simulink model "sim_sys2"  (R2013b)
settings: Solver=ode45  StartTime=0.0  StopTime=5000  RelTol=1e-3
undefined symbols (not defined in the file or in its folder): msdft_comb, resonator, sys_lib, twiddle_factors
libraries: xbsIndex_r4 x3996, casper_library_misc x310, xps_library x1
(part 5 of 46)

== system sim_sys2/Subsystem/resonator37 ==
  note: No estoy tan seguro
      | de este delay....
  din : Inport
  sync : Inport  Port=2
  rst : Inport  Port=3
  Delay{,1..2,4} (4 alike) : xbsIndex_r4/Delay  rst=off  infoeditControl=Selection of Reset will increase slice count due to use of real FFs and instead of SRLs  en=off  latency=1  dbl_ovrd=off  reg_retiming=off  block_type=delay
  Delay3 : xbsIndex_r4/Delay  rst=off  infoeditControl=Selection of Reset will increase slice count due to use of real FFs and instead of SRLs  en=off  latency=5  dbl_ovrd=off  reg_retiming=off  block_type=delay
  cmult : Subsystem  AncestorBlock=casper_library_multipliers/cmult  mask(cmult){n_bits_a=input_bitsize, bin_pt_a=input_frac, n_bits_b=twid_bitsize, bin_pt_b=twid_bitsize-2, n_bits_ab=input_bitsize+twid_bitsize+1, bin_pt_ab=input_frac+twid_bitsize-2, quantization=Truncate, overflow=Wrap, in_latency=0, mult_latency=3, add_latency=1, conv_latency=1, conjugated=off, async=off, pipelined_enable=on, multiplier_implementation=behavioral HDL}
      mask prompts: n_bits_a "Number of Bits 'a'"; bin_pt_a "Binary Point 'a'"; n_bits_b "Number of Bits 'b'"; bin_pt_b "Binary Point 'b'"; n_bits_ab "Number of Bits 'ab'"; bin_pt_ab "Binary Point 'ab'"; in_latency "Input latency"; mult_latency "Multiplier Latency"; add_latency "Adder Latency"; conv_latency "Convert latency"; conjugated "Conjugate"; async "asynchronous operation"; pipelined_enable "enable pipeline"; multiplier_implementation "Multiplier implementation"
      mask help:
      | Multiplies two complex numbers using 4 multipliers and 2 adders.
      | Conjugation is optional.
      mask init: same as sim_sys2/Subsystem/resonator/cmult
      settings: AttributesFormatString=|
      | 11_9 * 15_13 ==> 27_22
      | Truncate, Wrap
      | Latency=0
      mask TypeOptions quantization: Truncate | Round  (unbiased: +/- Inf) | Round  (unbiased: Even Values)
      mask TypeOptions overflow: Wrap | Saturate | Flag as error
      mask TypeOptions multiplier_implementation: behavioral HDL | standard core | embedded multiplier core
  complex_conj : Subsystem  AncestorBlock=casper_library_misc/complex_conj  mask(complex_conj){n_inputs=1, n_bits=twid_bitsize, bin_pt=twid_bitsize-2, latency=1, overflow=Wrap}
      mask prompts: n_inputs "number simultaneous inputs"; n_bits "input bitwidth"; bin_pt "input binary point"; overflow "overflow strategy"
      mask help: Finds the complex conjugate of complex inputs.
      mask init:
      | complex_conj_init(gcb, ...
      |     'n_inputs', n_inputs, ...
      |     'n_bits', n_bits, ...
      |     'bin_pt', bin_pt, ...
      |     'latency', latency, ...
      |     'overflow', overflow);
      mask TypeOptions overflow: Wrap | Saturate | Flag as error
  complex_sum : Subsystem  mask(complex_sum){a_bitsize=input_bitsize+twid_bitsize+1, a_frac=input_frac+twid_bitsize-2, b_bitsize=res_bitsize, b_frac=input_frac+twid_bitsize-2, out_bitsize=res_bitsize, latency=add_lat}
      mask prompts: out_bitsize "output_bitsize"
      mask init: same as sim_sys2/Subsystem/resonator/complex_sum
      settings: AttributesFormatString=latency=0
  twiddle : Subsystem  mask(msdft_twiddle_factors){fft_len=fft_len, bin_num=bin_number, twid_bitsize=twid_bitsize}
      mask prompts: fft_len "fft_len(2^)"; bin_num "bin number"; twid_bitsize "twiddle bitsize"
      mask init:
      | twid_msdft_init(gcb, ...
      |         'fft_len', fft_len, ...
      |         'bin_num', bin_num, ...
      |         'twid_bitsize', twid_bitsize)
      settings: AttributesFormatString=N=10, k=87
  Out1 : Outport
  twidd : Outport  Port=2
  wires:
  Delay4/1 -> twidd/1
  Delay3/1 -> Delay4/1
  Delay1/1 -> Delay3/1
  Delay2/1 -> complex_sum/2(b)
  complex_sum/1(dout) -> Out1/1, Delay2/1
  cmult/1(ab) -> complex_sum/1(a)
  Delay/1 -> cmult/1(a)
  complex_conj/1(z*) -> cmult/2(b)
  twiddle/1(dout) -> Delay1/1, complex_conj/1(z)
  din/1 -> Delay/1
  rst/1 -> twiddle/2(rst)
  sync/1 -> twiddle/1(sync)

== system sim_sys2/Subsystem/resonator38 ==
  note: No estoy tan seguro
      | de este delay....
  din : Inport
  sync : Inport  Port=2
  rst : Inport  Port=3
  Delay{,1..2,4} (4 alike) : xbsIndex_r4/Delay  rst=off  infoeditControl=Selection of Reset will increase slice count due to use of real FFs and instead of SRLs  en=off  latency=1  dbl_ovrd=off  reg_retiming=off  block_type=delay
  Delay3 : xbsIndex_r4/Delay  rst=off  infoeditControl=Selection of Reset will increase slice count due to use of real FFs and instead of SRLs  en=off  latency=5  dbl_ovrd=off  reg_retiming=off  block_type=delay
  cmult : Subsystem  AncestorBlock=casper_library_multipliers/cmult  mask(cmult){n_bits_a=input_bitsize, bin_pt_a=input_frac, n_bits_b=twid_bitsize, bin_pt_b=twid_bitsize-2, n_bits_ab=input_bitsize+twid_bitsize+1, bin_pt_ab=input_frac+twid_bitsize-2, quantization=Truncate, overflow=Wrap, in_latency=0, mult_latency=3, add_latency=1, conv_latency=1, conjugated=off, async=off, pipelined_enable=on, multiplier_implementation=behavioral HDL}
      mask prompts: n_bits_a "Number of Bits 'a'"; bin_pt_a "Binary Point 'a'"; n_bits_b "Number of Bits 'b'"; bin_pt_b "Binary Point 'b'"; n_bits_ab "Number of Bits 'ab'"; bin_pt_ab "Binary Point 'ab'"; in_latency "Input latency"; mult_latency "Multiplier Latency"; add_latency "Adder Latency"; conv_latency "Convert latency"; conjugated "Conjugate"; async "asynchronous operation"; pipelined_enable "enable pipeline"; multiplier_implementation "Multiplier implementation"
      mask help:
      | Multiplies two complex numbers using 4 multipliers and 2 adders.
      | Conjugation is optional.
      mask init: same as sim_sys2/Subsystem/resonator/cmult
      settings: AttributesFormatString=|
      | 11_9 * 15_13 ==> 27_22
      | Truncate, Wrap
      | Latency=0
      mask TypeOptions quantization: Truncate | Round  (unbiased: +/- Inf) | Round  (unbiased: Even Values)
      mask TypeOptions overflow: Wrap | Saturate | Flag as error
      mask TypeOptions multiplier_implementation: behavioral HDL | standard core | embedded multiplier core
  complex_conj : Subsystem  AncestorBlock=casper_library_misc/complex_conj  mask(complex_conj){n_inputs=1, n_bits=twid_bitsize, bin_pt=twid_bitsize-2, latency=1, overflow=Wrap}
      mask prompts: n_inputs "number simultaneous inputs"; n_bits "input bitwidth"; bin_pt "input binary point"; overflow "overflow strategy"
      mask help: Finds the complex conjugate of complex inputs.
      mask init:
      | complex_conj_init(gcb, ...
      |     'n_inputs', n_inputs, ...
      |     'n_bits', n_bits, ...
      |     'bin_pt', bin_pt, ...
      |     'latency', latency, ...
      |     'overflow', overflow);
      mask TypeOptions overflow: Wrap | Saturate | Flag as error
  complex_sum : Subsystem  mask(complex_sum){a_bitsize=input_bitsize+twid_bitsize+1, a_frac=input_frac+twid_bitsize-2, b_bitsize=res_bitsize, b_frac=input_frac+twid_bitsize-2, out_bitsize=res_bitsize, latency=add_lat}
      mask prompts: out_bitsize "output_bitsize"
      mask init: same as sim_sys2/Subsystem/resonator/complex_sum
      settings: AttributesFormatString=latency=0
  twiddle : Subsystem  mask(msdft_twiddle_factors){fft_len=fft_len, bin_num=bin_number, twid_bitsize=twid_bitsize}
      mask prompts: fft_len "fft_len(2^)"; bin_num "bin number"; twid_bitsize "twiddle bitsize"
      mask init:
      | twid_msdft_init(gcb, ...
      |         'fft_len', fft_len, ...
      |         'bin_num', bin_num, ...
      |         'twid_bitsize', twid_bitsize)
      settings: AttributesFormatString=N=10, k=88
  Out1 : Outport
  twidd : Outport  Port=2
  wires:
  Delay4/1 -> twidd/1
  Delay3/1 -> Delay4/1
  Delay1/1 -> Delay3/1
  Delay2/1 -> complex_sum/2(b)
  complex_sum/1(dout) -> Out1/1, Delay2/1
  cmult/1(ab) -> complex_sum/1(a)
  Delay/1 -> cmult/1(a)
  complex_conj/1(z*) -> cmult/2(b)
  twiddle/1(dout) -> Delay1/1, complex_conj/1(z)
  din/1 -> Delay/1
  rst/1 -> twiddle/2(rst)
  sync/1 -> twiddle/1(sync)

== system sim_sys2/Subsystem/resonator39 ==
  note: No estoy tan seguro
      | de este delay....
  din : Inport
  sync : Inport  Port=2
  rst : Inport  Port=3
  Delay{,1..2,4} (4 alike) : xbsIndex_r4/Delay  rst=off  infoeditControl=Selection of Reset will increase slice count due to use of real FFs and instead of SRLs  en=off  latency=1  dbl_ovrd=off  reg_retiming=off  block_type=delay
  Delay3 : xbsIndex_r4/Delay  rst=off  infoeditControl=Selection of Reset will increase slice count due to use of real FFs and instead of SRLs  en=off  latency=5  dbl_ovrd=off  reg_retiming=off  block_type=delay
  cmult : Subsystem  AncestorBlock=casper_library_multipliers/cmult  mask(cmult){n_bits_a=input_bitsize, bin_pt_a=input_frac, n_bits_b=twid_bitsize, bin_pt_b=twid_bitsize-2, n_bits_ab=input_bitsize+twid_bitsize+1, bin_pt_ab=input_frac+twid_bitsize-2, quantization=Truncate, overflow=Wrap, in_latency=0, mult_latency=3, add_latency=1, conv_latency=1, conjugated=off, async=off, pipelined_enable=on, multiplier_implementation=behavioral HDL}
      mask prompts: n_bits_a "Number of Bits 'a'"; bin_pt_a "Binary Point 'a'"; n_bits_b "Number of Bits 'b'"; bin_pt_b "Binary Point 'b'"; n_bits_ab "Number of Bits 'ab'"; bin_pt_ab "Binary Point 'ab'"; in_latency "Input latency"; mult_latency "Multiplier Latency"; add_latency "Adder Latency"; conv_latency "Convert latency"; conjugated "Conjugate"; async "asynchronous operation"; pipelined_enable "enable pipeline"; multiplier_implementation "Multiplier implementation"
      mask help:
      | Multiplies two complex numbers using 4 multipliers and 2 adders.
      | Conjugation is optional.
      mask init: same as sim_sys2/Subsystem/resonator/cmult
      settings: AttributesFormatString=|
      | 11_9 * 15_13 ==> 27_22
      | Truncate, Wrap
      | Latency=0
      mask TypeOptions quantization: Truncate | Round  (unbiased: +/- Inf) | Round  (unbiased: Even Values)
      mask TypeOptions overflow: Wrap | Saturate | Flag as error
      mask TypeOptions multiplier_implementation: behavioral HDL | standard core | embedded multiplier core
  complex_conj : Subsystem  AncestorBlock=casper_library_misc/complex_conj  mask(complex_conj){n_inputs=1, n_bits=twid_bitsize, bin_pt=twid_bitsize-2, latency=1, overflow=Wrap}
      mask prompts: n_inputs "number simultaneous inputs"; n_bits "input bitwidth"; bin_pt "input binary point"; overflow "overflow strategy"
      mask help: Finds the complex conjugate of complex inputs.
      mask init:
      | complex_conj_init(gcb, ...
      |     'n_inputs', n_inputs, ...
      |     'n_bits', n_bits, ...
      |     'bin_pt', bin_pt, ...
      |     'latency', latency, ...
      |     'overflow', overflow);
      mask TypeOptions overflow: Wrap | Saturate | Flag as error
  complex_sum : Subsystem  mask(complex_sum){a_bitsize=input_bitsize+twid_bitsize+1, a_frac=input_frac+twid_bitsize-2, b_bitsize=res_bitsize, b_frac=input_frac+twid_bitsize-2, out_bitsize=res_bitsize, latency=add_lat}
      mask prompts: out_bitsize "output_bitsize"
      mask init: same as sim_sys2/Subsystem/resonator/complex_sum
      settings: AttributesFormatString=latency=0
  twiddle : Subsystem  mask(msdft_twiddle_factors){fft_len=fft_len, bin_num=bin_number, twid_bitsize=twid_bitsize}
      mask prompts: fft_len "fft_len(2^)"; bin_num "bin number"; twid_bitsize "twiddle bitsize"
      mask init:
      | twid_msdft_init(gcb, ...
      |         'fft_len', fft_len, ...
      |         'bin_num', bin_num, ...
      |         'twid_bitsize', twid_bitsize)
      settings: AttributesFormatString=N=10, k=89
  Out1 : Outport
  twidd : Outport  Port=2
  wires:
  Delay4/1 -> twidd/1
  Delay3/1 -> Delay4/1
  Delay1/1 -> Delay3/1
  Delay2/1 -> complex_sum/2(b)
  complex_sum/1(dout) -> Out1/1, Delay2/1
  cmult/1(ab) -> complex_sum/1(a)
  Delay/1 -> cmult/1(a)
  complex_conj/1(z*) -> cmult/2(b)
  twiddle/1(dout) -> Delay1/1, complex_conj/1(z)
  din/1 -> Delay/1
  rst/1 -> twiddle/2(rst)
  sync/1 -> twiddle/1(sync)

== system sim_sys2/Subsystem/resonator4 ==
  note: No estoy tan seguro
      | de este delay....
  din : Inport
  sync : Inport  Port=2
  rst : Inport  Port=3
  Delay{,1..2,4} (4 alike) : xbsIndex_r4/Delay  rst=off  infoeditControl=Selection of Reset will increase slice count due to use of real FFs and instead of SRLs  en=off  latency=1  dbl_ovrd=off  reg_retiming=off  block_type=delay
  Delay3 : xbsIndex_r4/Delay  rst=off  infoeditControl=Selection of Reset will increase slice count due to use of real FFs and instead of SRLs  en=off  latency=5  dbl_ovrd=off  reg_retiming=off  block_type=delay
  cmult : Subsystem  AncestorBlock=casper_library_multipliers/cmult  mask(cmult){n_bits_a=input_bitsize, bin_pt_a=input_frac, n_bits_b=twid_bitsize, bin_pt_b=twid_bitsize-2, n_bits_ab=input_bitsize+twid_bitsize+1, bin_pt_ab=input_frac+twid_bitsize-2, quantization=Truncate, overflow=Wrap, in_latency=0, mult_latency=3, add_latency=1, conv_latency=1, conjugated=off, async=off, pipelined_enable=on, multiplier_implementation=behavioral HDL}
      mask prompts: n_bits_a "Number of Bits 'a'"; bin_pt_a "Binary Point 'a'"; n_bits_b "Number of Bits 'b'"; bin_pt_b "Binary Point 'b'"; n_bits_ab "Number of Bits 'ab'"; bin_pt_ab "Binary Point 'ab'"; in_latency "Input latency"; mult_latency "Multiplier Latency"; add_latency "Adder Latency"; conv_latency "Convert latency"; conjugated "Conjugate"; async "asynchronous operation"; pipelined_enable "enable pipeline"; multiplier_implementation "Multiplier implementation"
      mask help:
      | Multiplies two complex numbers using 4 multipliers and 2 adders.
      | Conjugation is optional.
      mask init: same as sim_sys2/Subsystem/resonator/cmult
      settings: AttributesFormatString=|
      | 11_9 * 15_13 ==> 27_22
      | Truncate, Wrap
      | Latency=0
      mask TypeOptions quantization: Truncate | Round  (unbiased: +/- Inf) | Round  (unbiased: Even Values)
      mask TypeOptions overflow: Wrap | Saturate | Flag as error
      mask TypeOptions multiplier_implementation: behavioral HDL | standard core | embedded multiplier core
  complex_conj : Subsystem  AncestorBlock=casper_library_misc/complex_conj  mask(complex_conj){n_inputs=1, n_bits=twid_bitsize, bin_pt=twid_bitsize-2, latency=1, overflow=Wrap}
      mask prompts: n_inputs "number simultaneous inputs"; n_bits "input bitwidth"; bin_pt "input binary point"; overflow "overflow strategy"
      mask help: Finds the complex conjugate of complex inputs.
      mask init:
      | complex_conj_init(gcb, ...
      |     'n_inputs', n_inputs, ...
      |     'n_bits', n_bits, ...
      |     'bin_pt', bin_pt, ...
      |     'latency', latency, ...
      |     'overflow', overflow);
      mask TypeOptions overflow: Wrap | Saturate | Flag as error
  complex_sum : Subsystem  mask(complex_sum){a_bitsize=input_bitsize+twid_bitsize+1, a_frac=input_frac+twid_bitsize-2, b_bitsize=res_bitsize, b_frac=input_frac+twid_bitsize-2, out_bitsize=res_bitsize, latency=add_lat}
      mask prompts: out_bitsize "output_bitsize"
      mask init: same as sim_sys2/Subsystem/resonator/complex_sum
      settings: AttributesFormatString=latency=0
  twiddle : Subsystem  mask(msdft_twiddle_factors){fft_len=fft_len, bin_num=bin_number, twid_bitsize=twid_bitsize}
      mask prompts: fft_len "fft_len(2^)"; bin_num "bin number"; twid_bitsize "twiddle bitsize"
      mask init:
      | twid_msdft_init(gcb, ...
      |         'fft_len', fft_len, ...
      |         'bin_num', bin_num, ...
      |         'twid_bitsize', twid_bitsize)
      settings: AttributesFormatString=N=10, k=54
  Out1 : Outport
  twidd : Outport  Port=2
  wires:
  Delay4/1 -> twidd/1
  Delay3/1 -> Delay4/1
  Delay1/1 -> Delay3/1
  Delay2/1 -> complex_sum/2(b)
  complex_sum/1(dout) -> Out1/1, Delay2/1
  cmult/1(ab) -> complex_sum/1(a)
  Delay/1 -> cmult/1(a)
  complex_conj/1(z*) -> cmult/2(b)
  twiddle/1(dout) -> Delay1/1, complex_conj/1(z)
  din/1 -> Delay/1
  rst/1 -> twiddle/2(rst)
  sync/1 -> twiddle/1(sync)

== system sim_sys2/Subsystem/resonator40 ==
  note: No estoy tan seguro
      | de este delay....
  din : Inport
  sync : Inport  Port=2
  rst : Inport  Port=3
  Delay{,1..2,4} (4 alike) : xbsIndex_r4/Delay  rst=off  infoeditControl=Selection of Reset will increase slice count due to use of real FFs and instead of SRLs  en=off  latency=1  dbl_ovrd=off  reg_retiming=off  block_type=delay
  Delay3 : xbsIndex_r4/Delay  rst=off  infoeditControl=Selection of Reset will increase slice count due to use of real FFs and instead of SRLs  en=off  latency=5  dbl_ovrd=off  reg_retiming=off  block_type=delay
  cmult : Subsystem  AncestorBlock=casper_library_multipliers/cmult  mask(cmult){n_bits_a=input_bitsize, bin_pt_a=input_frac, n_bits_b=twid_bitsize, bin_pt_b=twid_bitsize-2, n_bits_ab=input_bitsize+twid_bitsize+1, bin_pt_ab=input_frac+twid_bitsize-2, quantization=Truncate, overflow=Wrap, in_latency=0, mult_latency=3, add_latency=1, conv_latency=1, conjugated=off, async=off, pipelined_enable=on, multiplier_implementation=behavioral HDL}
      mask prompts: n_bits_a "Number of Bits 'a'"; bin_pt_a "Binary Point 'a'"; n_bits_b "Number of Bits 'b'"; bin_pt_b "Binary Point 'b'"; n_bits_ab "Number of Bits 'ab'"; bin_pt_ab "Binary Point 'ab'"; in_latency "Input latency"; mult_latency "Multiplier Latency"; add_latency "Adder Latency"; conv_latency "Convert latency"; conjugated "Conjugate"; async "asynchronous operation"; pipelined_enable "enable pipeline"; multiplier_implementation "Multiplier implementation"
      mask help:
      | Multiplies two complex numbers using 4 multipliers and 2 adders.
      | Conjugation is optional.
      mask init: same as sim_sys2/Subsystem/resonator/cmult
      settings: AttributesFormatString=|
      | 11_9 * 15_13 ==> 27_22
      | Truncate, Wrap
      | Latency=0
      mask TypeOptions quantization: Truncate | Round  (unbiased: +/- Inf) | Round  (unbiased: Even Values)
      mask TypeOptions overflow: Wrap | Saturate | Flag as error
      mask TypeOptions multiplier_implementation: behavioral HDL | standard core | embedded multiplier core
  complex_conj : Subsystem  AncestorBlock=casper_library_misc/complex_conj  mask(complex_conj){n_inputs=1, n_bits=twid_bitsize, bin_pt=twid_bitsize-2, latency=1, overflow=Wrap}
      mask prompts: n_inputs "number simultaneous inputs"; n_bits "input bitwidth"; bin_pt "input binary point"; overflow "overflow strategy"
      mask help: Finds the complex conjugate of complex inputs.
      mask init:
      | complex_conj_init(gcb, ...
      |     'n_inputs', n_inputs, ...
      |     'n_bits', n_bits, ...
      |     'bin_pt', bin_pt, ...
      |     'latency', latency, ...
      |     'overflow', overflow);
      mask TypeOptions overflow: Wrap | Saturate | Flag as error
  complex_sum : Subsystem  mask(complex_sum){a_bitsize=input_bitsize+twid_bitsize+1, a_frac=input_frac+twid_bitsize-2, b_bitsize=res_bitsize, b_frac=input_frac+twid_bitsize-2, out_bitsize=res_bitsize, latency=add_lat}
      mask prompts: out_bitsize "output_bitsize"
      mask init: same as sim_sys2/Subsystem/resonator/complex_sum
      settings: AttributesFormatString=latency=0
  twiddle : Subsystem  mask(msdft_twiddle_factors){fft_len=fft_len, bin_num=bin_number, twid_bitsize=twid_bitsize}
      mask prompts: fft_len "fft_len(2^)"; bin_num "bin number"; twid_bitsize "twiddle bitsize"
      mask init:
      | twid_msdft_init(gcb, ...
      |         'fft_len', fft_len, ...
      |         'bin_num', bin_num, ...
      |         'twid_bitsize', twid_bitsize)
      settings: AttributesFormatString=N=10, k=90
  Out1 : Outport
  twidd : Outport  Port=2
  wires:
  Delay4/1 -> twidd/1
  Delay3/1 -> Delay4/1
  Delay1/1 -> Delay3/1
  Delay2/1 -> complex_sum/2(b)
  complex_sum/1(dout) -> Out1/1, Delay2/1
  cmult/1(ab) -> complex_sum/1(a)
  Delay/1 -> cmult/1(a)
  complex_conj/1(z*) -> cmult/2(b)
  twiddle/1(dout) -> Delay1/1, complex_conj/1(z)
  din/1 -> Delay/1
  rst/1 -> twiddle/2(rst)
  sync/1 -> twiddle/1(sync)

== system sim_sys2/Subsystem/resonator41 ==
  note: No estoy tan seguro
      | de este delay....
  din : Inport
  sync : Inport  Port=2
  rst : Inport  Port=3
  Delay{,1..2,4} (4 alike) : xbsIndex_r4/Delay  rst=off  infoeditControl=Selection of Reset will increase slice count due to use of real FFs and instead of SRLs  en=off  latency=1  dbl_ovrd=off  reg_retiming=off  block_type=delay
  Delay3 : xbsIndex_r4/Delay  rst=off  infoeditControl=Selection of Reset will increase slice count due to use of real FFs and instead of SRLs  en=off  latency=5  dbl_ovrd=off  reg_retiming=off  block_type=delay
  cmult : Subsystem  AncestorBlock=casper_library_multipliers/cmult  mask(cmult){n_bits_a=input_bitsize, bin_pt_a=input_frac, n_bits_b=twid_bitsize, bin_pt_b=twid_bitsize-2, n_bits_ab=input_bitsize+twid_bitsize+1, bin_pt_ab=input_frac+twid_bitsize-2, quantization=Truncate, overflow=Wrap, in_latency=0, mult_latency=3, add_latency=1, conv_latency=1, conjugated=off, async=off, pipelined_enable=on, multiplier_implementation=behavioral HDL}
      mask prompts: n_bits_a "Number of Bits 'a'"; bin_pt_a "Binary Point 'a'"; n_bits_b "Number of Bits 'b'"; bin_pt_b "Binary Point 'b'"; n_bits_ab "Number of Bits 'ab'"; bin_pt_ab "Binary Point 'ab'"; in_latency "Input latency"; mult_latency "Multiplier Latency"; add_latency "Adder Latency"; conv_latency "Convert latency"; conjugated "Conjugate"; async "asynchronous operation"; pipelined_enable "enable pipeline"; multiplier_implementation "Multiplier implementation"
      mask help:
      | Multiplies two complex numbers using 4 multipliers and 2 adders.
      | Conjugation is optional.
      mask init: same as sim_sys2/Subsystem/resonator/cmult
      settings: AttributesFormatString=|
      | 11_9 * 15_13 ==> 27_22
      | Truncate, Wrap
      | Latency=0
      mask TypeOptions quantization: Truncate | Round  (unbiased: +/- Inf) | Round  (unbiased: Even Values)
      mask TypeOptions overflow: Wrap | Saturate | Flag as error
      mask TypeOptions multiplier_implementation: behavioral HDL | standard core | embedded multiplier core
  complex_conj : Subsystem  AncestorBlock=casper_library_misc/complex_conj  mask(complex_conj){n_inputs=1, n_bits=twid_bitsize, bin_pt=twid_bitsize-2, latency=1, overflow=Wrap}
      mask prompts: n_inputs "number simultaneous inputs"; n_bits "input bitwidth"; bin_pt "input binary point"; overflow "overflow strategy"
      mask help: Finds the complex conjugate of complex inputs.
      mask init:
      | complex_conj_init(gcb, ...
      |     'n_inputs', n_inputs, ...
      |     'n_bits', n_bits, ...
      |     'bin_pt', bin_pt, ...
      |     'latency', latency, ...
      |     'overflow', overflow);
      mask TypeOptions overflow: Wrap | Saturate | Flag as error
  complex_sum : Subsystem  mask(complex_sum){a_bitsize=input_bitsize+twid_bitsize+1, a_frac=input_frac+twid_bitsize-2, b_bitsize=res_bitsize, b_frac=input_frac+twid_bitsize-2, out_bitsize=res_bitsize, latency=add_lat}
      mask prompts: out_bitsize "output_bitsize"
      mask init: same as sim_sys2/Subsystem/resonator/complex_sum
      settings: AttributesFormatString=latency=0
  twiddle : Subsystem  mask(msdft_twiddle_factors){fft_len=fft_len, bin_num=bin_number, twid_bitsize=twid_bitsize}
      mask prompts: fft_len "fft_len(2^)"; bin_num "bin number"; twid_bitsize "twiddle bitsize"
      mask init:
      | twid_msdft_init(gcb, ...
      |         'fft_len', fft_len, ...
      |         'bin_num', bin_num, ...
      |         'twid_bitsize', twid_bitsize)
      settings: AttributesFormatString=N=10, k=91
  Out1 : Outport
  twidd : Outport  Port=2
  wires:
  Delay4/1 -> twidd/1
  Delay3/1 -> Delay4/1
  Delay1/1 -> Delay3/1
  Delay2/1 -> complex_sum/2(b)
  complex_sum/1(dout) -> Out1/1, Delay2/1
  cmult/1(ab) -> complex_sum/1(a)
  Delay/1 -> cmult/1(a)
  complex_conj/1(z*) -> cmult/2(b)
  twiddle/1(dout) -> Delay1/1, complex_conj/1(z)
  din/1 -> Delay/1
  rst/1 -> twiddle/2(rst)
  sync/1 -> twiddle/1(sync)

== system sim_sys2/Subsystem/resonator42 ==
  note: No estoy tan seguro
      | de este delay....
  din : Inport
  sync : Inport  Port=2
  rst : Inport  Port=3
  Delay{,1..2,4} (4 alike) : xbsIndex_r4/Delay  rst=off  infoeditControl=Selection of Reset will increase slice count due to use of real FFs and instead of SRLs  en=off  latency=1  dbl_ovrd=off  reg_retiming=off  block_type=delay
  Delay3 : xbsIndex_r4/Delay  rst=off  infoeditControl=Selection of Reset will increase slice count due to use of real FFs and instead of SRLs  en=off  latency=5  dbl_ovrd=off  reg_retiming=off  block_type=delay
  cmult : Subsystem  AncestorBlock=casper_library_multipliers/cmult  mask(cmult){n_bits_a=input_bitsize, bin_pt_a=input_frac, n_bits_b=twid_bitsize, bin_pt_b=twid_bitsize-2, n_bits_ab=input_bitsize+twid_bitsize+1, bin_pt_ab=input_frac+twid_bitsize-2, quantization=Truncate, overflow=Wrap, in_latency=0, mult_latency=3, add_latency=1, conv_latency=1, conjugated=off, async=off, pipelined_enable=on, multiplier_implementation=behavioral HDL}
      mask prompts: n_bits_a "Number of Bits 'a'"; bin_pt_a "Binary Point 'a'"; n_bits_b "Number of Bits 'b'"; bin_pt_b "Binary Point 'b'"; n_bits_ab "Number of Bits 'ab'"; bin_pt_ab "Binary Point 'ab'"; in_latency "Input latency"; mult_latency "Multiplier Latency"; add_latency "Adder Latency"; conv_latency "Convert latency"; conjugated "Conjugate"; async "asynchronous operation"; pipelined_enable "enable pipeline"; multiplier_implementation "Multiplier implementation"
      mask help:
      | Multiplies two complex numbers using 4 multipliers and 2 adders.
      | Conjugation is optional.
      mask init: same as sim_sys2/Subsystem/resonator/cmult
      settings: AttributesFormatString=|
      | 11_9 * 15_13 ==> 27_22
      | Truncate, Wrap
      | Latency=0
      mask TypeOptions quantization: Truncate | Round  (unbiased: +/- Inf) | Round  (unbiased: Even Values)
      mask TypeOptions overflow: Wrap | Saturate | Flag as error
      mask TypeOptions multiplier_implementation: behavioral HDL | standard core | embedded multiplier core
  complex_conj : Subsystem  AncestorBlock=casper_library_misc/complex_conj  mask(complex_conj){n_inputs=1, n_bits=twid_bitsize, bin_pt=twid_bitsize-2, latency=1, overflow=Wrap}
      mask prompts: n_inputs "number simultaneous inputs"; n_bits "input bitwidth"; bin_pt "input binary point"; overflow "overflow strategy"
      mask help: Finds the complex conjugate of complex inputs.
      mask init:
      | complex_conj_init(gcb, ...
      |     'n_inputs', n_inputs, ...
      |     'n_bits', n_bits, ...
      |     'bin_pt', bin_pt, ...
      |     'latency', latency, ...
      |     'overflow', overflow);
      mask TypeOptions overflow: Wrap | Saturate | Flag as error
  complex_sum : Subsystem  mask(complex_sum){a_bitsize=input_bitsize+twid_bitsize+1, a_frac=input_frac+twid_bitsize-2, b_bitsize=res_bitsize, b_frac=input_frac+twid_bitsize-2, out_bitsize=res_bitsize, latency=add_lat}
      mask prompts: out_bitsize "output_bitsize"
      mask init: same as sim_sys2/Subsystem/resonator/complex_sum
      settings: AttributesFormatString=latency=0
  twiddle : Subsystem  mask(msdft_twiddle_factors){fft_len=fft_len, bin_num=bin_number, twid_bitsize=twid_bitsize}
      mask prompts: fft_len "fft_len(2^)"; bin_num "bin number"; twid_bitsize "twiddle bitsize"
      mask init:
      | twid_msdft_init(gcb, ...
      |         'fft_len', fft_len, ...
      |         'bin_num', bin_num, ...
      |         'twid_bitsize', twid_bitsize)
      settings: AttributesFormatString=N=10, k=92
  Out1 : Outport
  twidd : Outport  Port=2
  wires:
  Delay4/1 -> twidd/1
  Delay3/1 -> Delay4/1
  Delay1/1 -> Delay3/1
  Delay2/1 -> complex_sum/2(b)
  complex_sum/1(dout) -> Out1/1, Delay2/1
  cmult/1(ab) -> complex_sum/1(a)
  Delay/1 -> cmult/1(a)
  complex_conj/1(z*) -> cmult/2(b)
  twiddle/1(dout) -> Delay1/1, complex_conj/1(z)
  din/1 -> Delay/1
  rst/1 -> twiddle/2(rst)
  sync/1 -> twiddle/1(sync)

== system sim_sys2/Subsystem/resonator43 ==
  note: No estoy tan seguro
      | de este delay....
  din : Inport
  sync : Inport  Port=2
  rst : Inport  Port=3
  Delay{,1..2,4} (4 alike) : xbsIndex_r4/Delay  rst=off  infoeditControl=Selection of Reset will increase slice count due to use of real FFs and instead of SRLs  en=off  latency=1  dbl_ovrd=off  reg_retiming=off  block_type=delay
  Delay3 : xbsIndex_r4/Delay  rst=off  infoeditControl=Selection of Reset will increase slice count due to use of real FFs and instead of SRLs  en=off  latency=5  dbl_ovrd=off  reg_retiming=off  block_type=delay
  cmult : Subsystem  AncestorBlock=casper_library_multipliers/cmult  mask(cmult){n_bits_a=input_bitsize, bin_pt_a=input_frac, n_bits_b=twid_bitsize, bin_pt_b=twid_bitsize-2, n_bits_ab=input_bitsize+twid_bitsize+1, bin_pt_ab=input_frac+twid_bitsize-2, quantization=Truncate, overflow=Wrap, in_latency=0, mult_latency=3, add_latency=1, conv_latency=1, conjugated=off, async=off, pipelined_enable=on, multiplier_implementation=behavioral HDL}
      mask prompts: n_bits_a "Number of Bits 'a'"; bin_pt_a "Binary Point 'a'"; n_bits_b "Number of Bits 'b'"; bin_pt_b "Binary Point 'b'"; n_bits_ab "Number of Bits 'ab'"; bin_pt_ab "Binary Point 'ab'"; in_latency "Input latency"; mult_latency "Multiplier Latency"; add_latency "Adder Latency"; conv_latency "Convert latency"; conjugated "Conjugate"; async "asynchronous operation"; pipelined_enable "enable pipeline"; multiplier_implementation "Multiplier implementation"
      mask help:
      | Multiplies two complex numbers using 4 multipliers and 2 adders.
      | Conjugation is optional.
      mask init: same as sim_sys2/Subsystem/resonator/cmult
      settings: AttributesFormatString=|
      | 11_9 * 15_13 ==> 27_22
      | Truncate, Wrap
      | Latency=0
      mask TypeOptions quantization: Truncate | Round  (unbiased: +/- Inf) | Round  (unbiased: Even Values)
      mask TypeOptions overflow: Wrap | Saturate | Flag as error
      mask TypeOptions multiplier_implementation: behavioral HDL | standard core | embedded multiplier core
  complex_conj : Subsystem  AncestorBlock=casper_library_misc/complex_conj  mask(complex_conj){n_inputs=1, n_bits=twid_bitsize, bin_pt=twid_bitsize-2, latency=1, overflow=Wrap}
      mask prompts: n_inputs "number simultaneous inputs"; n_bits "input bitwidth"; bin_pt "input binary point"; overflow "overflow strategy"
      mask help: Finds the complex conjugate of complex inputs.
      mask init:
      | complex_conj_init(gcb, ...
      |     'n_inputs', n_inputs, ...
      |     'n_bits', n_bits, ...
      |     'bin_pt', bin_pt, ...
      |     'latency', latency, ...
      |     'overflow', overflow);
      mask TypeOptions overflow: Wrap | Saturate | Flag as error
  complex_sum : Subsystem  mask(complex_sum){a_bitsize=input_bitsize+twid_bitsize+1, a_frac=input_frac+twid_bitsize-2, b_bitsize=res_bitsize, b_frac=input_frac+twid_bitsize-2, out_bitsize=res_bitsize, latency=add_lat}
      mask prompts: out_bitsize "output_bitsize"
      mask init: same as sim_sys2/Subsystem/resonator/complex_sum
      settings: AttributesFormatString=latency=0
  twiddle : Subsystem  mask(msdft_twiddle_factors){fft_len=fft_len, bin_num=bin_number, twid_bitsize=twid_bitsize}
      mask prompts: fft_len "fft_len(2^)"; bin_num "bin number"; twid_bitsize "twiddle bitsize"
      mask init:
      | twid_msdft_init(gcb, ...
      |         'fft_len', fft_len, ...
      |         'bin_num', bin_num, ...
      |         'twid_bitsize', twid_bitsize)
      settings: AttributesFormatString=N=10, k=93
  Out1 : Outport
  twidd : Outport  Port=2
  wires:
  Delay4/1 -> twidd/1
  Delay3/1 -> Delay4/1
  Delay1/1 -> Delay3/1
  Delay2/1 -> complex_sum/2(b)
  complex_sum/1(dout) -> Out1/1, Delay2/1
  cmult/1(ab) -> complex_sum/1(a)
  Delay/1 -> cmult/1(a)
  complex_conj/1(z*) -> cmult/2(b)
  twiddle/1(dout) -> Delay1/1, complex_conj/1(z)
  din/1 -> Delay/1
  rst/1 -> twiddle/2(rst)
  sync/1 -> twiddle/1(sync)

== system sim_sys2/Subsystem/resonator44 ==
  note: No estoy tan seguro
      | de este delay....
  din : Inport
  sync : Inport  Port=2
  rst : Inport  Port=3
  Delay{,1..2,4} (4 alike) : xbsIndex_r4/Delay  rst=off  infoeditControl=Selection of Reset will increase slice count due to use of real FFs and instead of SRLs  en=off  latency=1  dbl_ovrd=off  reg_retiming=off  block_type=delay
  Delay3 : xbsIndex_r4/Delay  rst=off  infoeditControl=Selection of Reset will increase slice count due to use of real FFs and instead of SRLs  en=off  latency=5  dbl_ovrd=off  reg_retiming=off  block_type=delay
  cmult : Subsystem  AncestorBlock=casper_library_multipliers/cmult  mask(cmult){n_bits_a=input_bitsize, bin_pt_a=input_frac, n_bits_b=twid_bitsize, bin_pt_b=twid_bitsize-2, n_bits_ab=input_bitsize+twid_bitsize+1, bin_pt_ab=input_frac+twid_bitsize-2, quantization=Truncate, overflow=Wrap, in_latency=0, mult_latency=3, add_latency=1, conv_latency=1, conjugated=off, async=off, pipelined_enable=on, multiplier_implementation=behavioral HDL}
      mask prompts: n_bits_a "Number of Bits 'a'"; bin_pt_a "Binary Point 'a'"; n_bits_b "Number of Bits 'b'"; bin_pt_b "Binary Point 'b'"; n_bits_ab "Number of Bits 'ab'"; bin_pt_ab "Binary Point 'ab'"; in_latency "Input latency"; mult_latency "Multiplier Latency"; add_latency "Adder Latency"; conv_latency "Convert latency"; conjugated "Conjugate"; async "asynchronous operation"; pipelined_enable "enable pipeline"; multiplier_implementation "Multiplier implementation"
      mask help:
      | Multiplies two complex numbers using 4 multipliers and 2 adders.
      | Conjugation is optional.
      mask init: same as sim_sys2/Subsystem/resonator/cmult
      settings: AttributesFormatString=|
      | 11_9 * 15_13 ==> 27_22
      | Truncate, Wrap
      | Latency=0
      mask TypeOptions quantization: Truncate | Round  (unbiased: +/- Inf) | Round  (unbiased: Even Values)
      mask TypeOptions overflow: Wrap | Saturate | Flag as error
      mask TypeOptions multiplier_implementation: behavioral HDL | standard core | embedded multiplier core
  complex_conj : Subsystem  AncestorBlock=casper_library_misc/complex_conj  mask(complex_conj){n_inputs=1, n_bits=twid_bitsize, bin_pt=twid_bitsize-2, latency=1, overflow=Wrap}
      mask prompts: n_inputs "number simultaneous inputs"; n_bits "input bitwidth"; bin_pt "input binary point"; overflow "overflow strategy"
      mask help: Finds the complex conjugate of complex inputs.
      mask init:
      | complex_conj_init(gcb, ...
      |     'n_inputs', n_inputs, ...
      |     'n_bits', n_bits, ...
      |     'bin_pt', bin_pt, ...
      |     'latency', latency, ...
      |     'overflow', overflow);
      mask TypeOptions overflow: Wrap | Saturate | Flag as error
  complex_sum : Subsystem  mask(complex_sum){a_bitsize=input_bitsize+twid_bitsize+1, a_frac=input_frac+twid_bitsize-2, b_bitsize=res_bitsize, b_frac=input_frac+twid_bitsize-2, out_bitsize=res_bitsize, latency=add_lat}
      mask prompts: out_bitsize "output_bitsize"
      mask init: same as sim_sys2/Subsystem/resonator/complex_sum
      settings: AttributesFormatString=latency=0
  twiddle : Subsystem  mask(msdft_twiddle_factors){fft_len=fft_len, bin_num=bin_number, twid_bitsize=twid_bitsize}
      mask prompts: fft_len "fft_len(2^)"; bin_num "bin number"; twid_bitsize "twiddle bitsize"
      mask init:
      | twid_msdft_init(gcb, ...
      |         'fft_len', fft_len, ...
      |         'bin_num', bin_num, ...
      |         'twid_bitsize', twid_bitsize)
      settings: AttributesFormatString=N=10, k=94
  Out1 : Outport
  twidd : Outport  Port=2
  wires:
  Delay4/1 -> twidd/1
  Delay3/1 -> Delay4/1
  Delay1/1 -> Delay3/1
  Delay2/1 -> complex_sum/2(b)
  complex_sum/1(dout) -> Out1/1, Delay2/1
  cmult/1(ab) -> complex_sum/1(a)
  Delay/1 -> cmult/1(a)
  complex_conj/1(z*) -> cmult/2(b)
  twiddle/1(dout) -> Delay1/1, complex_conj/1(z)
  din/1 -> Delay/1
  rst/1 -> twiddle/2(rst)
  sync/1 -> twiddle/1(sync)

== system sim_sys2/Subsystem/resonator45 ==
  note: No estoy tan seguro
      | de este delay....
  din : Inport
  sync : Inport  Port=2
  rst : Inport  Port=3
  Delay{,1..2,4} (4 alike) : xbsIndex_r4/Delay  rst=off  infoeditControl=Selection of Reset will increase slice count due to use of real FFs and instead of SRLs  en=off  latency=1  dbl_ovrd=off  reg_retiming=off  block_type=delay
  Delay3 : xbsIndex_r4/Delay  rst=off  infoeditControl=Selection of Reset will increase slice count due to use of real FFs and instead of SRLs  en=off  latency=5  dbl_ovrd=off  reg_retiming=off  block_type=delay
  cmult : Subsystem  AncestorBlock=casper_library_multipliers/cmult  mask(cmult){n_bits_a=input_bitsize, bin_pt_a=input_frac, n_bits_b=twid_bitsize, bin_pt_b=twid_bitsize-2, n_bits_ab=input_bitsize+twid_bitsize+1, bin_pt_ab=input_frac+twid_bitsize-2, quantization=Truncate, overflow=Wrap, in_latency=0, mult_latency=3, add_latency=1, conv_latency=1, conjugated=off, async=off, pipelined_enable=on, multiplier_implementation=behavioral HDL}
      mask prompts: n_bits_a "Number of Bits 'a'"; bin_pt_a "Binary Point 'a'"; n_bits_b "Number of Bits 'b'"; bin_pt_b "Binary Point 'b'"; n_bits_ab "Number of Bits 'ab'"; bin_pt_ab "Binary Point 'ab'"; in_latency "Input latency"; mult_latency "Multiplier Latency"; add_latency "Adder Latency"; conv_latency "Convert latency"; conjugated "Conjugate"; async "asynchronous operation"; pipelined_enable "enable pipeline"; multiplier_implementation "Multiplier implementation"
      mask help:
      | Multiplies two complex numbers using 4 multipliers and 2 adders.
      | Conjugation is optional.
      mask init: same as sim_sys2/Subsystem/resonator/cmult
      settings: AttributesFormatString=|
      | 11_9 * 15_13 ==> 27_22
      | Truncate, Wrap
      | Latency=0
      mask TypeOptions quantization: Truncate | Round  (unbiased: +/- Inf) | Round  (unbiased: Even Values)
      mask TypeOptions overflow: Wrap | Saturate | Flag as error
      mask TypeOptions multiplier_implementation: behavioral HDL | standard core | embedded multiplier core
  complex_conj : Subsystem  AncestorBlock=casper_library_misc/complex_conj  mask(complex_conj){n_inputs=1, n_bits=twid_bitsize, bin_pt=twid_bitsize-2, latency=1, overflow=Wrap}
      mask prompts: n_inputs "number simultaneous inputs"; n_bits "input bitwidth"; bin_pt "input binary point"; overflow "overflow strategy"
      mask help: Finds the complex conjugate of complex inputs.
      mask init:
      | complex_conj_init(gcb, ...
      |     'n_inputs', n_inputs, ...
      |     'n_bits', n_bits, ...
      |     'bin_pt', bin_pt, ...
      |     'latency', latency, ...
      |     'overflow', overflow);
      mask TypeOptions overflow: Wrap | Saturate | Flag as error
  complex_sum : Subsystem  mask(complex_sum){a_bitsize=input_bitsize+twid_bitsize+1, a_frac=input_frac+twid_bitsize-2, b_bitsize=res_bitsize, b_frac=input_frac+twid_bitsize-2, out_bitsize=res_bitsize, latency=add_lat}
      mask prompts: out_bitsize "output_bitsize"
      mask init: same as sim_sys2/Subsystem/resonator/complex_sum
      settings: AttributesFormatString=latency=0
  twiddle : Subsystem  mask(msdft_twiddle_factors){fft_len=fft_len, bin_num=bin_number, twid_bitsize=twid_bitsize}
      mask prompts: fft_len "fft_len(2^)"; bin_num "bin number"; twid_bitsize "twiddle bitsize"
      mask init:
      | twid_msdft_init(gcb, ...
      |         'fft_len', fft_len, ...
      |         'bin_num', bin_num, ...
      |         'twid_bitsize', twid_bitsize)
      settings: AttributesFormatString=N=10, k=95
  Out1 : Outport
  twidd : Outport  Port=2
  wires:
  Delay4/1 -> twidd/1
  Delay3/1 -> Delay4/1
  Delay1/1 -> Delay3/1
  Delay2/1 -> complex_sum/2(b)
  complex_sum/1(dout) -> Out1/1, Delay2/1
  cmult/1(ab) -> complex_sum/1(a)
  Delay/1 -> cmult/1(a)
  complex_conj/1(z*) -> cmult/2(b)
  twiddle/1(dout) -> Delay1/1, complex_conj/1(z)
  din/1 -> Delay/1
  rst/1 -> twiddle/2(rst)
  sync/1 -> twiddle/1(sync)

== system sim_sys2/Subsystem/resonator46 ==
  note: No estoy tan seguro
      | de este delay....
  din : Inport
  sync : Inport  Port=2
  rst : Inport  Port=3
  Delay{,1..2,4} (4 alike) : xbsIndex_r4/Delay  rst=off  infoeditControl=Selection of Reset will increase slice count due to use of real FFs and instead of SRLs  en=off  latency=1  dbl_ovrd=off  reg_retiming=off  block_type=delay
  Delay3 : xbsIndex_r4/Delay  rst=off  infoeditControl=Selection of Reset will increase slice count due to use of real FFs and instead of SRLs  en=off  latency=5  dbl_ovrd=off  reg_retiming=off  block_type=delay
  cmult : Subsystem  AncestorBlock=casper_library_multipliers/cmult  mask(cmult){n_bits_a=input_bitsize, bin_pt_a=input_frac, n_bits_b=twid_bitsize, bin_pt_b=twid_bitsize-2, n_bits_ab=input_bitsize+twid_bitsize+1, bin_pt_ab=input_frac+twid_bitsize-2, quantization=Truncate, overflow=Wrap, in_latency=0, mult_latency=3, add_latency=1, conv_latency=1, conjugated=off, async=off, pipelined_enable=on, multiplier_implementation=behavioral HDL}
      mask prompts: n_bits_a "Number of Bits 'a'"; bin_pt_a "Binary Point 'a'"; n_bits_b "Number of Bits 'b'"; bin_pt_b "Binary Point 'b'"; n_bits_ab "Number of Bits 'ab'"; bin_pt_ab "Binary Point 'ab'"; in_latency "Input latency"; mult_latency "Multiplier Latency"; add_latency "Adder Latency"; conv_latency "Convert latency"; conjugated "Conjugate"; async "asynchronous operation"; pipelined_enable "enable pipeline"; multiplier_implementation "Multiplier implementation"
      mask help:
      | Multiplies two complex numbers using 4 multipliers and 2 adders.
      | Conjugation is optional.
      mask init: same as sim_sys2/Subsystem/resonator/cmult
      settings: AttributesFormatString=|
      | 11_9 * 15_13 ==> 27_22
      | Truncate, Wrap
      | Latency=0
      mask TypeOptions quantization: Truncate | Round  (unbiased: +/- Inf) | Round  (unbiased: Even Values)
      mask TypeOptions overflow: Wrap | Saturate | Flag as error
      mask TypeOptions multiplier_implementation: behavioral HDL | standard core | embedded multiplier core
  complex_conj : Subsystem  AncestorBlock=casper_library_misc/complex_conj  mask(complex_conj){n_inputs=1, n_bits=twid_bitsize, bin_pt=twid_bitsize-2, latency=1, overflow=Wrap}
      mask prompts: n_inputs "number simultaneous inputs"; n_bits "input bitwidth"; bin_pt "input binary point"; overflow "overflow strategy"
      mask help: Finds the complex conjugate of complex inputs.
      mask init:
      | complex_conj_init(gcb, ...
      |     'n_inputs', n_inputs, ...
      |     'n_bits', n_bits, ...
      |     'bin_pt', bin_pt, ...
      |     'latency', latency, ...
      |     'overflow', overflow);
      mask TypeOptions overflow: Wrap | Saturate | Flag as error
  complex_sum : Subsystem  mask(complex_sum){a_bitsize=input_bitsize+twid_bitsize+1, a_frac=input_frac+twid_bitsize-2, b_bitsize=res_bitsize, b_frac=input_frac+twid_bitsize-2, out_bitsize=res_bitsize, latency=add_lat}
      mask prompts: out_bitsize "output_bitsize"
      mask init: same as sim_sys2/Subsystem/resonator/complex_sum
      settings: AttributesFormatString=latency=0
  twiddle : Subsystem  mask(msdft_twiddle_factors){fft_len=fft_len, bin_num=bin_number, twid_bitsize=twid_bitsize}
      mask prompts: fft_len "fft_len(2^)"; bin_num "bin number"; twid_bitsize "twiddle bitsize"
      mask init:
      | twid_msdft_init(gcb, ...
      |         'fft_len', fft_len, ...
      |         'bin_num', bin_num, ...
      |         'twid_bitsize', twid_bitsize)
      settings: AttributesFormatString=N=10, k=96
  Out1 : Outport
  twidd : Outport  Port=2
  wires:
  Delay4/1 -> twidd/1
  Delay3/1 -> Delay4/1
  Delay1/1 -> Delay3/1
  Delay2/1 -> complex_sum/2(b)
  complex_sum/1(dout) -> Out1/1, Delay2/1
  cmult/1(ab) -> complex_sum/1(a)
  Delay/1 -> cmult/1(a)
  complex_conj/1(z*) -> cmult/2(b)
  twiddle/1(dout) -> Delay1/1, complex_conj/1(z)
  din/1 -> Delay/1
  rst/1 -> twiddle/2(rst)
  sync/1 -> twiddle/1(sync)

== system sim_sys2/Subsystem/resonator47 ==
  note: No estoy tan seguro
      | de este delay....
  din : Inport
  sync : Inport  Port=2
  rst : Inport  Port=3
  Delay{,1..2,4} (4 alike) : xbsIndex_r4/Delay  rst=off  infoeditControl=Selection of Reset will increase slice count due to use of real FFs and instead of SRLs  en=off  latency=1  dbl_ovrd=off  reg_retiming=off  block_type=delay
  Delay3 : xbsIndex_r4/Delay  rst=off  infoeditControl=Selection of Reset will increase slice count due to use of real FFs and instead of SRLs  en=off  latency=5  dbl_ovrd=off  reg_retiming=off  block_type=delay
  cmult : Subsystem  AncestorBlock=casper_library_multipliers/cmult  mask(cmult){n_bits_a=input_bitsize, bin_pt_a=input_frac, n_bits_b=twid_bitsize, bin_pt_b=twid_bitsize-2, n_bits_ab=input_bitsize+twid_bitsize+1, bin_pt_ab=input_frac+twid_bitsize-2, quantization=Truncate, overflow=Wrap, in_latency=0, mult_latency=3, add_latency=1, conv_latency=1, conjugated=off, async=off, pipelined_enable=on, multiplier_implementation=behavioral HDL}
      mask prompts: n_bits_a "Number of Bits 'a'"; bin_pt_a "Binary Point 'a'"; n_bits_b "Number of Bits 'b'"; bin_pt_b "Binary Point 'b'"; n_bits_ab "Number of Bits 'ab'"; bin_pt_ab "Binary Point 'ab'"; in_latency "Input latency"; mult_latency "Multiplier Latency"; add_latency "Adder Latency"; conv_latency "Convert latency"; conjugated "Conjugate"; async "asynchronous operation"; pipelined_enable "enable pipeline"; multiplier_implementation "Multiplier implementation"
      mask help:
      | Multiplies two complex numbers using 4 multipliers and 2 adders.
      | Conjugation is optional.
      mask init: same as sim_sys2/Subsystem/resonator/cmult
      settings: AttributesFormatString=|
      | 11_9 * 15_13 ==> 27_22
      | Truncate, Wrap
      | Latency=0
      mask TypeOptions quantization: Truncate | Round  (unbiased: +/- Inf) | Round  (unbiased: Even Values)
      mask TypeOptions overflow: Wrap | Saturate | Flag as error
      mask TypeOptions multiplier_implementation: behavioral HDL | standard core | embedded multiplier core
  complex_conj : Subsystem  AncestorBlock=casper_library_misc/complex_conj  mask(complex_conj){n_inputs=1, n_bits=twid_bitsize, bin_pt=twid_bitsize-2, latency=1, overflow=Wrap}
      mask prompts: n_inputs "number simultaneous inputs"; n_bits "input bitwidth"; bin_pt "input binary point"; overflow "overflow strategy"
      mask help: Finds the complex conjugate of complex inputs.
      mask init:
      | complex_conj_init(gcb, ...
      |     'n_inputs', n_inputs, ...
      |     'n_bits', n_bits, ...
      |     'bin_pt', bin_pt, ...
      |     'latency', latency, ...
      |     'overflow', overflow);
      mask TypeOptions overflow: Wrap | Saturate | Flag as error
  complex_sum : Subsystem  mask(complex_sum){a_bitsize=input_bitsize+twid_bitsize+1, a_frac=input_frac+twid_bitsize-2, b_bitsize=res_bitsize, b_frac=input_frac+twid_bitsize-2, out_bitsize=res_bitsize, latency=add_lat}
      mask prompts: out_bitsize "output_bitsize"
      mask init: same as sim_sys2/Subsystem/resonator/complex_sum
      settings: AttributesFormatString=latency=0
  twiddle : Subsystem  mask(msdft_twiddle_factors){fft_len=fft_len, bin_num=bin_number, twid_bitsize=twid_bitsize}
      mask prompts: fft_len "fft_len(2^)"; bin_num "bin number"; twid_bitsize "twiddle bitsize"
      mask init:
      | twid_msdft_init(gcb, ...
      |         'fft_len', fft_len, ...
      |         'bin_num', bin_num, ...
      |         'twid_bitsize', twid_bitsize)
      settings: AttributesFormatString=N=10, k=97
  Out1 : Outport
  twidd : Outport  Port=2
  wires:
  Delay4/1 -> twidd/1
  Delay3/1 -> Delay4/1
  Delay1/1 -> Delay3/1
  Delay2/1 -> complex_sum/2(b)
  complex_sum/1(dout) -> Out1/1, Delay2/1
  cmult/1(ab) -> complex_sum/1(a)
  Delay/1 -> cmult/1(a)
  complex_conj/1(z*) -> cmult/2(b)
  twiddle/1(dout) -> Delay1/1, complex_conj/1(z)
  din/1 -> Delay/1
  rst/1 -> twiddle/2(rst)
  sync/1 -> twiddle/1(sync)
